simulink model "Multibody_2modules"  (R2024a)
settings: Solver=FixedStepAuto  StartTime=0.0  StopTime=TF  FixedStep=Ts  RelTol=1e-3
InitFcn:
  | close all
  | kinematics_2_modules
StopFcn:
  | results
model workspace: external: MATLAB File C:\Users\ricar\Documentos\MATLAB\OMNI_COUPLED\Coupled_SIMSCAPE_DataFile.m (data not in the file)
values from neighbouring files (symbols this model uses):
  eje_1 = 1    [kinematics_2_modules.m]    (also in kinematics_3_modules.m; kinematics_4modules.m; kinematics_front.m)
  eje_2 = 1    [kinematics_2_modules.m]    (also in kinematics_3_modules.m; kinematics_4modules.m; kinematics_front.m)
  eje_3 = 1    [kinematics_2_modules.m]    (also in kinematics_3_modules.m; kinematics_4modules.m; kinematics_front.m)
  eje_4 = 1    [kinematics_2_modules.m]    (also in kinematics_3_modules.m; kinematics_4modules.m; kinematics_front.m)
undefined symbols (not defined in the file or in its folder): fun_2mod_DK, smiData, X, Y, Z
libraries: sm_lib x362, nesl_utility x17, simulink x4, dspsigops x1
(part 1 of 6)
settings Model: Creator=ricar  LastModifiedBy=ricar
settings OptimizationCC: ReuseModelBlockBuffer=off
settings RTWCC: GPUComputeCapability=3.5
settings ExplorerConfigSet: InternalSimMechanicsExplorerSettings="<ExplorerConfiguration><canonicalview>planar_xy</canonicalview><AnimationSetting><BasePlaybackSpeed>1.0</BasePlaybackSpeed><PlaybackSpeedFactor>1.0</PlaybackSpeedFactor></AnimationSetting><TilePanel><TileInfo><Tiles Columns=\"1\" Count=\"1\" Rows=\"1\"><Column Weight=\"1\"/><Row Weight=\"1\"/><Tile Height=\"1\" Width=\"1\" X=\"0\" Y=\"0\"/></Tiles></TileInfo><SceneInfo><SceneViewer><BGColor><R>0.60000002384185791</R><G>0.60000002384185791</G><B>0.60000002384185791</B></BGColor><Camera><DoPerspective>off</DoPerspective><Position><X>1.22678896204454646</X><Y>1.20628904029276285</Y><Z>1.22678906359187656</Z></Position><Center><X>2.53292032547855483e-08</X><Y>-0.0204998964225804117</Y><Z>1.26876533262237912e-07</Z></Center><Up><X>-0.408248290463863073</X><Y>0.816496580927726145</Y><Z>-0.408248290463863073</Z></Up><ViewLimDist>1</ViewLimDist><YLim>1.38972711630507817</YLim><XLim>2.18495985507965074</XLim></Camera></SceneViewer></SceneInfo></TilePanel><MechEditorPanel><Cameras/><GfxPanelCameraMap/><VideoCreator><PlaybackSpeedRatio>1.0</PlaybackSpeedRatio><FrameRate>30</FrameRate><VideoFormat>Motion JPEG AVI</VideoFormat><FrameSize>auto</FrameSize></VideoCreator></MechEditorPanel></ExplorerConfiguration>"

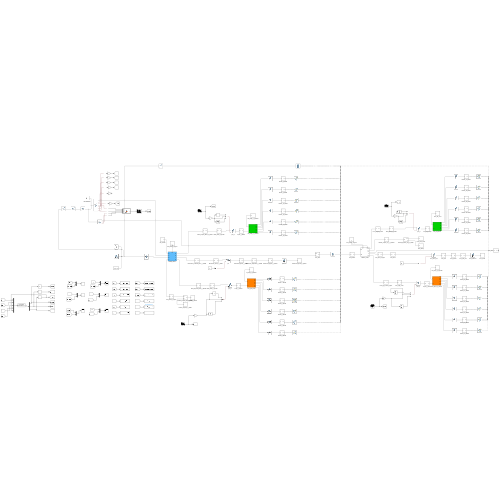
[thumbnail: Simulink's stored preview of the top-level diagram]
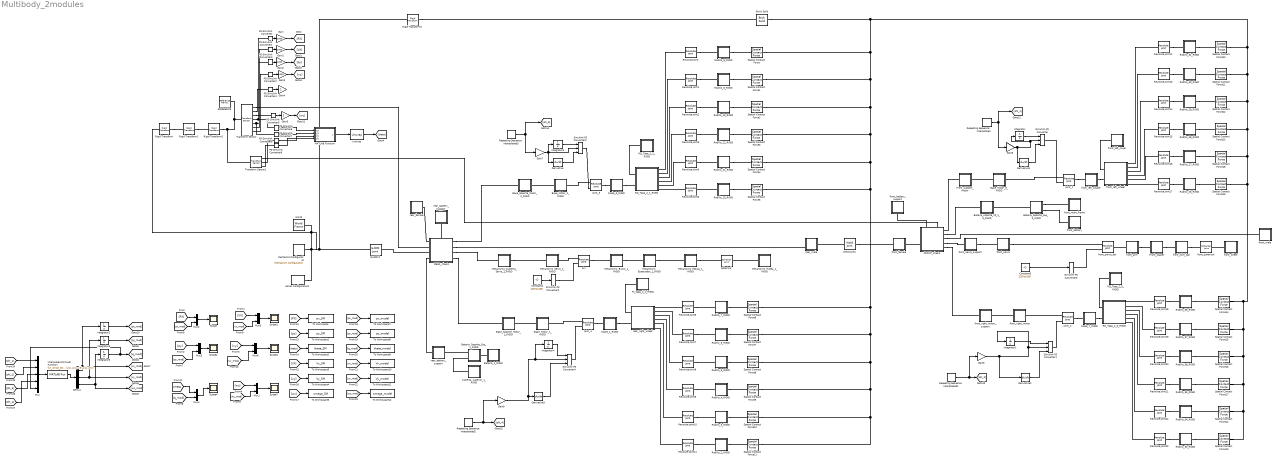
== system Multibody_2modules ==
  Base_Motor_1_RIGID : Subsystem
  Base_Motor_2_RIGID : Subsystem
  Base_Motor_6_RIGID : Subsystem
  Base_Soporte_Motor_1_RIGID : Subsystem
  Base_Soporte_Motor_2_RIGID : Subsystem
  Bateria_1_RIGID : Subsystem
  Bateria_Soporte_Sup_1_RIGID : Subsystem
  Bateria_Soporte_Sup_3_RIGID : Subsystem
  Bateria_soporte_Inf_1_3_RIGID : Subsystem
  Brick Solid : sm_lib/Body Elements/Brick Solid  BrickDimensions=[3 .002 3]  BrickDimensionsUnits=m  ExportEntireGeometry=on  InertiaType=CalculateFromGeometry  BasedOnType=Density  Density=1000  DensityUnits=kg/m^3  Mass=1  MassUnits=kg  CenterOfMass=[0 0 0]  CenterOfMassUnits=m  MomentsOfInertia=[1 1 1]  MomentsOfInertiaUnits=kg*m^2  ProductsOfInertia=[0 0 0]  ProductsOfInertiaUnits=kg*m^2  GraphicType=FromGeometry  MarkerShape=Sphere  MarkerSize=10  GraphicVisPropType=SimpleVisualProperties  GraphicDiffuseColor=[1 .6 .6]  GraphicOpacity=1  GraphicSpecularColor=[0.5 0.5 0.5 1.0]  GraphicAmbientColor=[0.15 0.15 0.15 1.0]  GraphicEmissiveColor=[0.0 0.0 0.0 1.0]  GraphicShininess=75  DoExposeReferenceFrame=on  SerializedFrames=<Frames/>
  Constant4 : Constant  Value=225*pi/180
  Constant5 : Constant  Value=225*pi/180
  Cople_1_RIGID : Subsystem
  Cople_3_RIGID : Subsystem
  Cople_7_RIGID : Subsystem
  Demux : Demux  Outputs=3
  Derivative{,1..3} (4 alike) : Derivative
  FRONT_chasis : Subsystem
      settings: PortSchema="{\"entries\":[{\"content\":{\"sides\":[{\"content\":{\"connectorIds\":[\"LConn1\",\"LConn2\"]},\"type\":\"ConnectorPlacement.EquallySpacedRectSide\",\"uuid\":\"2f193958-adda-4ec1-9c1e-8d18e10a43bf\"},{\"content\":{\"connectorIds\":[\"RConn1\",\"RConn2\",\"RConn3\",\"RConn4\",\"RConn5\"],\"side\":\"RIGHT\"},\"type\":\"ConnectorPlacement.EquallySpacedRectSide\",\"uuid\":\"9da4c68d-326e-4e0f-8b14-dbca64ff3e46\"},{\"content\":{\"connectorIds\":[\"LConn3\",\"LConn4\"],\"side\":\"TOP\"},\"type\":\"ConnectorPlacement.EquallySpacedRectSide\",\"uuid\":\"282e500d-48cf-43b0-8f8a-0690bc1d8b4d\"},{\"content\":{\"side\":\"BOTTOM\"},\"type\":\"ConnectorPlacement.EquallySpacedRectSide\",\"uuid\":\"3772ac25-9249-4303-a1a7-4471353d0084\"}]},\"type\":\"ConnectorPlacement.EquallySpacedConnector\",\"uuid\":\"3fae074b-7e70-469c-9f21-d7560799185b\"}],\"packageUris\":[\"http://schema.mathworks.com/mf0/Connector/R2020b\"],\"version\":\"1.0\"}"
  Front_spacer : Subsystem
  Front_support_motor : Subsystem
  Gain{,1..3} (4 alike) : Gain  Gain=1000
  Gain4 : Gain
  Gain5 : Gain
  Gain6 : Gain  Gain=eje_1
  Gain7 : Gain  Gain=eje_3
  Gain8 : Gain  Gain=eje_2
  Gain9 : Gain  Gain=eje_4
  Integrator{,1..6} (7 alike) : Integrator
  Interpreted MATLAB Function : MATLABFcn  MATLABFcn=fun_2mod_DK(u(1),u(2),u(3),u(4),u(5))
  MATLAB Function : MATLAB Function  TreatAsAtomicUnit=on
  Mecanismo_Brazo_1_RIGID : Subsystem
  Mecanismo_Cubierta_Servo_1_RIGID : Subsystem
  Mecanismo_Espaciador_1_RIGID : Subsystem
  Mecanismo_Rptula_1_RIGID : Subsystem
  Mecanismo_Rueda_1_RIGID : Subsystem
  Mecanismo_Servo_1_RIGID : Subsystem
  MechanismConfiguration : sm_lib/Utilities/Mechanism Configuration  UniformGravity=Constant  GravityVector=[0 -9.80665 0]  GravityVectorUnits=m/s^2  LinearizationDelta=0.001  JointModeTransitionNonlinearIterations=2
  Mux : Mux  Inputs=5
  Mux{1..6} (6 alike) : Mux  Inputs=2
  PS-Simulink Converter{,1..9} (10 alike) : nesl_utility/PS-Simulink Converter  PhysicalDomain=network_engine_domain  SubClassName=ps_output  LeftPortType=input  RightPortType=output  PseudoPeriodic=off  Frequencies=[]  VectorFormat=inherit  Unit=inherit  AffineConversion=off
  RD_Tapa_2_1_RIGID : Subsystem
  RD_Tapa_2_2_RIGID : Subsystem
  RD_Tapa_2_5_RIGID : Subsystem
  RD_Tapa_2_6_RIGID : Subsystem
  REAR_chasis : Subsystem
      settings: PortSchema="{\"entries\":[{\"content\":{\"sides\":[{\"content\":{\"connectorIds\":[\"LConn1\",\"LConn2\",\"LConn3\",\"LConn4\"]},\"type\":\"ConnectorPlacement.EquallySpacedRectSide\",\"uuid\":\"2f193958-adda-4ec1-9c1e-8d18e10a43bf\"},{\"content\":{\"connectorIds\":[\"RConn1\",\"RConn2\",\"RConn3\",\"RConn4\"],\"side\":\"RIGHT\"},\"type\":\"ConnectorPlacement.EquallySpacedRectSide\",\"uuid\":\"9da4c68d-326e-4e0f-8b14-dbca64ff3e46\"},{\"content\":{\"connectorIds\":[\"LConn5\"],\"side\":\"TOP\"},\"type\":\"ConnectorPlacement.EquallySpacedRectSide\",\"uuid\":\"282e500d-48cf-43b0-8f8a-0690bc1d8b4d\"}]},\"type\":\"ConnectorPlacement.EquallySpacedConnector\",\"uuid\":\"3fae074b-7e70-469c-9f21-d7560799185b\"}],\"packageUris\":[\"http://schema.mathworks.com/mf0/Connector/R2020b\"],\"version\":\"1.0\"}"
  REFERENCE : sm_lib/Frames and Transforms/Reference Frame
  RI_tapa_2_2_RIGID : Subsystem
  Repeating Sequence Interpolated : simulink/Sources/Repeating Sequence Interpolated  OutValues="1.5*[0  -1.49  -1.49  0   1.48  1.48   0  -2.96  -2.96  0  -1.46  -1.46 0]'"  TimeValues=[0 1 4 5 6 9 10 11 14 15 16 19 20]'  LookUpMeth=Interpolation-Use End Values  tsamp=0.0005  OutMin=[]  OutMax=[]  OutDataTypeStr=double  OutputDataTypeScalingMode=double  OutDataType=fixdt(0,8)  OutScaling=2^-10
  Repeating Sequence Interpolated1 : simulink/Sources/Repeating Sequence Interpolated  OutValues="1.5*[0  -1.49  -1.49  0  -4.44 -4.44   0  -2.96  -2.96  0  -1.46  -1.46 0]'"  TimeValues=[0 1 4 5 6 9 10 11 14 15 16 19 20]'  LookUpMeth=Interpolation-Use End Values  tsamp=0.0005  OutMin=[]  OutMax=[]  OutDataTypeStr=double  OutputDataTypeScalingMode=double  OutDataType=fixdt(0,8)  OutScaling=2^-10
  Repeating Sequence Interpolated2 : simulink/Sources/Repeating Sequence Interpolated  OutValues="1.5*[0   4.42   4.42  0  -1.48 -1.48   0   2.96   2.96  0  -1.49  -1.46 0]'"  TimeValues=[0 1 4 5 6 9 10 11 14 15 16 19 20]'  LookUpMeth=Interpolation-Use End Values  tsamp=0.0005  OutMin=[]  OutMax=[]  OutDataTypeStr=double  OutputDataTypeScalingMode=double  OutDataType=fixdt(0,8)  OutScaling=2^-10
  Repeating Sequence Interpolated3 : simulink/Sources/Repeating Sequence Interpolated  OutValues="1.5*[0   4.42   4.42  0   4.44  4.44   0   2.96   2.96  0  -1.46  -1.46 0]'"  TimeValues=[0 1 4 5 6 9 10 11 14 15 16 19 20]'  LookUpMeth=Interpolation-Use End Values  tsamp=0.0005  OutMin=[]  OutMax=[]  OutDataTypeStr=double  OutputDataTypeScalingMode=double  OutDataType=fixdt(0,8)  OutScaling=2^-10
  Revolute Joint{,1..23} (24 alike) : sm_lib/Joints/Revolute Joint  JointMode=Normal  CompositeWrenchDir=FollowerOnBase  CompositeWrenchFrame=BaseFrame  SenseConstraintForce=off  SenseConstraintTorque=off  SenseTotalForce=off  SenseTotalTorque=off  PositionTargetSpecify=off  PositionTargetPriority=High  PositionTargetValue=0  PositionTargetValueUnits=deg  VelocityTargetSpecify=off  VelocityTargetPriority=High  VelocityTargetValue=0  VelocityTargetValueUnits=deg/s  EquilibriumPosition=0  EquilibriumPositionUnits=deg  SpringStiffness=0  SpringStiffnessUnits=N*m/deg  DampingCoefficient=0  DampingCoefficientUnits=N*m/(deg/s)  LowerLimitSpecify=off  LowerLimitBound=-90  LowerLimitBoundUnits=deg  LowerLimitStiffness=1e4  LowerLimitStiffnessUnits=N*m/deg  LowerLimitDamping=10  LowerLimitDampingUnits=N*m/(deg/s)  LowerLimitTransitionRegionWidth=0.1  LowerLimitTransitionRegionWidthUnits=deg  UpperLimitSpecify=off  UpperLimitBound=90  UpperLimitBoundUnits=deg  UpperLimitStiffness=1e4  UpperLimitStiffnessUnits=N*m/deg  UpperLimitDamping=10  UpperLimitDampingUnits=N*m/(deg/s)  UpperLimitTransitionRegionWidth=0.1  UpperLimitTransitionRegionWidthUnits=deg  TorqueActuationMode=NoTorque  MotionActuationMode=ComputedMotion  SensePosition=off  SenseVelocity=off  SenseAcceleration=off  SenseTorqueForce=off  SenseLowerLimitTorqueForce=off  SenseUpperLimitTorqueForce=off
  Rigid Transform : sm_lib/Frames and Transforms/Rigid Transform  RotationMethod=StandardAxis  FollAlignAxisA=+X  BaseAlignAxisA=+Y  FollAlignAxisB=+Y  BaseAlignAxisB=+Z  RotationStandardAxis=+X  RotationAngle=-90  RotationAngleUnits=deg  RotationArbitraryAxis=[0 0 1]  RotationSequenceAxes=FollowerAxes  RotationSequence=XYX  RotationSequenceAngles=[0 0 0]  RotationSequenceAnglesUnits=deg  RotationMatrix=[1 0 0; 0 1 0; 0 0 1]  Quaternion=[1 0 0 0]  TranslationMethod=None  TranslationCartesianOffset=[0 0 0]  TranslationCartesianOffsetUnits=m  TranslationStandardAxis=+Z  TranslationStandardOffset=0  TranslationStandardOffsetUnits=m  TranslationROffset=0  TranslationROffsetUnits=m  TranslationThetaOffset=0  TranslationThetaOffsetUnits=deg  TranslationZOffset=0  TranslationZOffsetUnits=m
  Rigid Transform1 : sm_lib/Frames and Transforms/Rigid Transform  RotationMethod=StandardAxis  FollAlignAxisA=+X  BaseAlignAxisA=+Y  FollAlignAxisB=+Y  BaseAlignAxisB=+Z  RotationStandardAxis=+Z  RotationAngle=0  RotationAngleUnits=deg  RotationArbitraryAxis=[0 0 1]  RotationSequenceAxes=FollowerAxes  RotationSequence=XYX  RotationSequenceAngles=[0 0 0]  RotationSequenceAnglesUnits=deg  RotationMatrix=[1 0 0; 0 1 0; 0 0 1]  Quaternion=[1 0 0 0]  TranslationMethod=None  TranslationCartesianOffset=[0 0 0]  TranslationCartesianOffsetUnits=m  TranslationStandardAxis=+Z  TranslationStandardOffset=0  TranslationStandardOffsetUnits=m  TranslationROffset=0  TranslationROffsetUnits=m  TranslationThetaOffset=0  TranslationThetaOffsetUnits=deg  TranslationZOffset=0  TranslationZOffsetUnits=m
  Rigid Transform2 : sm_lib/Frames and Transforms/Rigid Transform  RotationMethod=None  FollAlignAxisA=+X  BaseAlignAxisA=+Y  FollAlignAxisB=+Y  BaseAlignAxisB=+Z  RotationStandardAxis=+Z  RotationAngle=0.0  RotationAngleUnits=deg  RotationArbitraryAxis=[0 0 1]  RotationSequenceAxes=FollowerAxes  RotationSequence=XYX  RotationSequenceAngles=[0 0 0]  RotationSequenceAnglesUnits=deg  RotationMatrix=[1 0 0; 0 1 0; 0 0 1]  Quaternion=[1 0 0 0]  TranslationMethod=StandardAxis  TranslationCartesianOffset=[0 0 0]  TranslationCartesianOffsetUnits=mm  TranslationStandardAxis=+X  TranslationStandardOffset=96-66  TranslationStandardOffsetUnits=mm  TranslationROffset=0  TranslationROffsetUnits=m  TranslationThetaOffset=0  TranslationThetaOffsetUnits=deg  TranslationZOffset=0  TranslationZOffsetUnits=m
  Rigid Transform3 : sm_lib/Frames and Transforms/Rigid Transform  RotationMethod=None  FollAlignAxisA=+X  BaseAlignAxisA=+Y  FollAlignAxisB=+Y  BaseAlignAxisB=+Z  RotationStandardAxis=+Z  RotationAngle=0  RotationAngleUnits=deg  RotationArbitraryAxis=[0 0 1]  RotationSequenceAxes=FollowerAxes  RotationSequence=XYX  RotationSequenceAngles=[0 0 0]  RotationSequenceAnglesUnits=deg  RotationMatrix=[1 0 0;0 1 0;0 0 1]  Quaternion=[1 0 0 0]  TranslationMethod=StandardAxis  TranslationCartesianOffset=[0 0 0]  TranslationCartesianOffsetUnits=m  TranslationStandardAxis=+Y  TranslationStandardOffset=-.0205  TranslationStandardOffsetUnits=m  TranslationROffset=0  TranslationROffsetUnits=m  TranslationThetaOffset=0  TranslationThetaOffsetUnits=deg  TranslationZOffset=0  TranslationZOffsetUnits=m
  Rodillo_10_RIGID : Subsystem
  Rodillo_11_RIGID : Subsystem
  Rodillo_12_RIGID : Subsystem
  Rodillo_13_RIGID : Subsystem
  Rodillo_26_RIGID : Subsystem
  Rodillo_27_RIGID : Subsystem
  Rodillo_28_RIGID : Subsystem
  Rodillo_29_RIGID : Subsystem
  Rodillo_2_RIGID : Subsystem
  Rodillo_30_RIGID : Subsystem
  Rodillo_31_RIGID : Subsystem
  Rodillo_33_RIGID : Subsystem
  Rodillo_34_RIGID : Subsystem
  Rodillo_35_RIGID : Subsystem
  Rodillo_36_RIGID : Subsystem
  Rodillo_37_RIGID : Subsystem
  Rodillo_38_RIGID : Subsystem
  Rodillo_3_RIGID : Subsystem
  Rodillo_4_RIGID : Subsystem
  Rodillo_5_RIGID : Subsystem
  Rodillo_6_RIGID : Subsystem
  Rodillo_7_RIGID : Subsystem
  Rodillo_8_RIGID : Subsystem
  Rodillo_9_RIGID : Subsystem
  Scope{,1..4,7} (6 alike) : Scope
  Simulink-PS Converter{,1,3..4} (4 alike) : nesl_utility/Simulink-PS Converter  PhysicalDomain=network_engine_domain  SubClassName=ps_input  LeftPortType=input  RightPortType=output  PseudoPeriodic=off  Frequencies=[]  NoiseDistribution=none  NoiseParameters=[]  Unit=1  AffineConversion=off  FilteringAndDerivatives=provide  SimscapeFilterOrder=1  InputFilterTimeConstant=0.001  UdotUserProvided=2
  Simulink-PS Converter2 : nesl_utility/Simulink-PS Converter  PhysicalDomain=network_engine_domain  SubClassName=ps_input  LeftPortType=input  RightPortType=output  PseudoPeriodic=off  Frequencies=[]  NoiseDistribution=none  NoiseParameters=[]  Unit=1  AffineConversion=off  FilteringAndDerivatives=zero  SimscapeFilterOrder=1  InputFilterTimeConstant=0.001  UdotUserProvided=0
  Simulink-PS Converter5 : nesl_utility/Simulink-PS Converter  PhysicalDomain=network_engine_domain  SubClassName=ps_input  LeftPortType=input  RightPortType=output  PseudoPeriodic=off  Frequencies=[]  NoiseDistribution=none  NoiseParameters=[]  Unit=1  AffineConversion=off  FilteringAndDerivatives=zero  SimscapeFilterOrder=1  InputFilterTimeConstant=0.001  UdotUserProvided=0
  SixDOF1 : sm_lib/Joints/6-DOF Joint  JointMode=Normal  CompositeWrenchDir=FollowerOnBase  CompositeWrenchFrame=BaseFrame  SenseConstraintForce=off  SenseConstraintTorque=off  SenseTotalForce=off  SenseTotalTorque=off  PxPositionTargetSpecify=off  PxPositionTargetPriority=High  PxPositionTargetValue=0  PxPositionTargetValueUnits=m  PxVelocityTargetSpecify=off  PxVelocityTargetPriority=High  PxVelocityTargetValue=0  PxVelocityTargetValueUnits=m/s  PxEquilibriumPosition=0  PxEquilibriumPositionUnits=m  PxSpringStiffness=0  PxSpringStiffnessUnits=N/m  PxDampingCoefficient=0  PxDampingCoefficientUnits=N/(m/s)  PxLowerLimitSpecify=off  PxLowerLimitBound=-1  PxLowerLimitBoundUnits=m  PxLowerLimitStiffness=1e6  PxLowerLimitStiffnessUnits=N/m  PxLowerLimitDamping=1e3  PxLowerLimitDampingUnits=N/(m/s)  PxLowerLimitTransitionRegionWidth=1e-4  PxLowerLimitTransitionRegionWidthUnits=m  PxUpperLimitSpecify=off  PxUpperLimitBound=1  PxUpperLimitBoundUnits=m  PxUpperLimitStiffness=1e6  PxUpperLimitStiffnessUnits=N/m  PxUpperLimitDamping=1e3  PxUpperLimitDampingUnits=N/(m/s)  PxUpperLimitTransitionRegionWidth=1e-4  PxUpperLimitTransitionRegionWidthUnits=m  PxTorqueActuationMode=NoTorque  PxMotionActuationMode=ComputedMotion  PxSensePosition=off  PxSenseVelocity=off  PxSenseAcceleration=off  PxSenseTorqueForce=off  PxSenseLowerLimitTorqueForce=off  PxSenseUpperLimitTorqueForce=off  PyPositionTargetSpecify=off  PyPositionTargetPriority=High  PyPositionTargetValue=0  PyPositionTargetValueUnits=m  PyVelocityTargetSpecify=off  PyVelocityTargetPriority=High  PyVelocityTargetValue=0  PyVelocityTargetValueUnits=m/s  PyEquilibriumPosition=0  PyEquilibriumPositionUnits=m  PySpringStiffness=0  PySpringStiffnessUnits=N/m  PyDampingCoefficient=0  PyDampingCoefficientUnits=N/(m/s)  PyLowerLimitSpecify=off  PyLowerLimitBound=-1  PyLowerLimitBoundUnits=m  PyLowerLimitStiffness=1e6  PyLowerLimitStiffnessUnits=N/m  PyLowerLimitDamping=1e3  PyLowerLimitDampingUnits=N/(m/s)  PyLowerLimitTransitionRegionWidth=1e-4  PyLowerLimitTransitionRegionWidthUnits=m  PyUpperLimitSpecify=off  PyUpperLimitBound=1  PyUpperLimitBoundUnits=m  PyUpperLimitStiffness=1e6  PyUpperLimitStiffnessUnits=N/m  PyUpperLimitDamping=1e3  PyUpperLimitDampingUnits=N/(m/s)  PyUpperLimitTransitionRegionWidth=1e-4  PyUpperLimitTransitionRegionWidthUnits=m  PyTorqueActuationMode=NoTorque  PyMotionActuationMode=ComputedMotion  PySensePosition=off  PySenseVelocity=off  PySenseAcceleration=off  PySenseTorqueForce=off  PySenseLowerLimitTorqueForce=off  PySenseUpperLimitTorqueForce=off  PzPositionTargetSpecify=off  PzPositionTargetPriority=High  PzPositionTargetValue=0  PzPositionTargetValueUnits=m  PzVelocityTargetSpecify=off  PzVelocityTargetPriority=High  PzVelocityTargetValue=0  PzVelocityTargetValueUnits=m/s  PzEquilibriumPosition=0  PzEquilibriumPositionUnits=m  PzSpringStiffness=0  PzSpringStiffnessUnits=N/m  PzDampingCoefficient=0  PzDampingCoefficientUnits=N/(m/s)  PzLowerLimitSpecify=off  PzLowerLimitBound=-1  PzLowerLimitBoundUnits=m  PzLowerLimitStiffness=1e6  PzLowerLimitStiffnessUnits=N/m  PzLowerLimitDamping=1e3  PzLowerLimitDampingUnits=N/(m/s)  PzLowerLimitTransitionRegionWidth=1e-4  PzLowerLimitTransitionRegionWidthUnits=m  PzUpperLimitSpecify=off  PzUpperLimitBound=1  PzUpperLimitBoundUnits=m  PzUpperLimitStiffness=1e6  PzUpperLimitStiffnessUnits=N/m  PzUpperLimitDamping=1e3  PzUpperLimitDampingUnits=N/(m/s)  PzUpperLimitTransitionRegionWidth=1e-4  PzUpperLimitTransitionRegionWidthUnits=m  PzTorqueActuationMode=NoTorque  PzMotionActuationMode=ComputedMotion  PzSensePosition=off  PzSenseVelocity=off  PzSenseAcceleration=off  PzSenseTorqueForce=off  PzSenseLowerLimitTorqueForce=off  PzSenseUpperLimitTorqueForce=off  SphPositionTargetSpecify=off  SphPositionTargetPriority=High  SphPositionTargetRotationMethod=None  SphPositionTargetFollAlignAxisA=+X  SphPositionTargetBaseAlignAxisA=+Y  SphPositionTargetFollAlignAxisB=+Y  SphPositionTargetBaseAlignAxisB=+Z  SphPositionTargetRotationStandardAxis=+Z  SphPositionTargetRotationAngle=0.0  SphPositionTargetRotationAngleUnits=deg  SphPositionTargetRotationArbitraryAxis=[0 0 1]  SphPositionTargetRotationSequenceAxes=FollowerAxes  SphPositionTargetRotationSequence=XYX  SphPositionTargetRotationSequenceAngles=[0 0 0]  SphPositionTargetRotationSequenceAnglesUnits=deg  SphPositionTargetRotationMatrix=[1 0 0; 0 1 0; 0 0 1]  SphPositionTargetQuaternion=[1 0 0 0]  SphVelocityTargetSpecify=off  SphVelocityTargetPriority=High  SphVelocityTargetValue=[0 0 0]  SphVelocityTargetValueUnits=deg/s  SphVelocityTargetInFollowerFrame=on  SphEqPosRotationMethod=None  SphEqPosFollAlignAxisA=+X  SphEqPosBaseAlignAxisA=+Y  SphEqPosFollAlignAxisB=+Y  SphEqPosBaseAlignAxisB=+Z  SphEqPosRotationStandardAxis=+Z  SphEqPosRotationAngle=0.0  SphEqPosRotationAngleUnits=deg  SphEqPosRotationArbitraryAxis=[0 0 1]  SphEqPosRotationSequenceAxes=FollowerAxes  SphEqPosRotationSequence=XYX  SphEqPosRotationSequenceAngles=[0 0 0]  SphEqPosRotationSequenceAnglesUnits=deg  SphEqPosRotationMatrix=[1 0 0; 0 1 0; 0 0 1]  SphEqPosQuaternion=[1 0 0 0]  SphSpringStiffness=0  SphSpringStiffnessUnits=N*m/deg  SphDampingCoefficient=0  SphDampingCoefficientUnits=N*m/(deg/s)  SphLowerLimitSpecify=off  SphLowerLimitBound=15  SphLowerLimitBoundUnits=deg  SphLowerLimitStiffness=1e4  SphLowerLimitStiffnessUnits=N*m/deg  SphLowerLimitDamping=10  SphLowerLimitDampingUnits=N*m/(deg/s)  SphLowerLimitTransitionRegionWidth=0.1  SphLowerLimitTransitionRegionWidthUnits=deg  SphUpperLimitSpecify=off  SphUpperLimitBound=45  SphUpperLimitBoundUnits=deg  SphUpperLimitStiffness=1e4  SphUpperLimitStiffnessUnits=N*m/deg  SphUpperLimitDamping=10  SphUpperLimitDampingUnits=N*m/(deg/s)  SphUpperLimitTransitionRegionWidth=0.1  SphUpperLimitTransitionRegionWidthUnits=deg  SphTorqueActuationMode=NoTorque  SphActuateTorqueX=off  SphActuateTorqueY=off  SphActuateTorqueZ=off  SphActuateTorque=off  SphActuationFrame=BaseFrame  SphSensePosition=off  SphSenseVelocityX=off  SphSenseVelocityY=off  SphSenseVelocityZ=off  SphSenseVelocity=off  SphSenseAccelerationX=off  SphSenseAccelerationY=off  SphSenseAccelerationZ=off  SphSenseAcceleration=off  SphSenseLowerLimitTorqueMag=off  SphSenseUpperLimitTorqueMag=off  SphSensingFrame=FollowerFrame
  Solver Configuration1 : nesl_utility/Solver Configuration  PhysicalDomain=network_engine_domain  SubClassName=solver  LeftPortType=input  RightPortType=generic  Tones=[]  Harmonics=[]  SimulateNoise=off  Profile=off  UseLocalSampling=off  EnableSwitchedLinearOptims=on  FrequencyDomain=off  UseCCode=off  RelTol=0.001  AbsTol=0.001  MinStep=1e-09  ToWorkspace=off  RevertToSquareIcSolve=off  NumHomotopyIterations=100  PhasorMode=off  PhasorModeNumHarmonics=1  ConsistencySolver=NEWTON_XTOL_AFTER_FTOL  IndexReductionMethod=DerivativeReplacement  DoDC=off  ResidualTolerance=1e-09  ConsistencyTolSource=GLOBAL  ConsistencyAbsTol=0.001  ConsistencyRelTol=0.001  ConsistencyTolFactor=0.001  UseLocalSolver=off  LocalSolverChoice=NE_BACKWARD_EULER_ADVANCER  ResolveIndetEquations=on  FunctionEvalNumThread=1  LocalSolverSampleTime=0.001  DoFixedCost=off  MaxNonlinIter=3  MaxModeIter=2  ComputeImpulses=off  ImpulseIterations=2  LinearAlgebra=auto  LinearAlgebraNumThread=0  EquationFormulation=NE_TIME_EF  DelaysMemoryBudget=1024  AutomaticFiltering=on  FilteringTimeConstant=0.001  PartitionStorageMethod=AS_NEEDED  PartitionMemoryBudget=1024  PartitionMethod=ROBUST  MultibodyUseLocalSolver=off  MultibodyLocalSolverChoice=ODE1  MultibodyLocalSolverSampleTime=0.001
  Spatial Contact Force{,1..23} (24 alike) : sm_lib/Forces and Torques/Spatial Contact Force  NormalForceType=SmoothSpringDamper  NormalStiffness=1e6  NormalStiffnessUnits=N/m  NormalDamping=1e3  NormalDampingUnits=N/(m/s)  NormalTransitionRegionWidth=1e-4  NormalTransitionRegionWidthUnits=m  FrictionType=SmoothStickSlip  CoefficientOfStaticFriction=0.5  CoefficientOfDynamicFriction=0.3  FrictionalCriticalVelocity=1e-3  FrictionalCriticalVelocityUnits=m/s  SenseContactSignal=off  SensePenetrationDepth=off  SenseSeparationDistance=off  SenseNormalForceMagnitude=off  SenseFrictionalForceMagnitude=off  SenseNormalVelocity=off  SenseTangentialVelocity=off  SenseContactBaseRotation=off  SenseContactBaseTranslation=off  SenseContactFollowerRotation=off  SenseContactFollowerTranslation=off  ZeroCrossDetectContactStartAndEnd=off
  Spherical : sm_lib/Joints/Spherical Joint  JointMode=Normal  CompositeWrenchDir=FollowerOnBase  CompositeWrenchFrame=BaseFrame  SenseConstraintForce=off  SenseConstraintTorque=off  SenseTotalForce=off  SenseTotalTorque=off  PositionTargetSpecify=off  PositionTargetPriority=Low  PositionTargetRotationMethod=ArbitraryAxis  PositionTargetFollAlignAxisA=+X  PositionTargetBaseAlignAxisA=+Y  PositionTargetFollAlignAxisB=+Y  PositionTargetBaseAlignAxisB=+Z  PositionTargetRotationStandardAxis=+Z  PositionTargetRotationAngle=smiData.SphericalJoint(1).S.Pos.Angle  PositionTargetRotationAngleUnits=deg  PositionTargetRotationArbitraryAxis=smiData.SphericalJoint(1).S.Pos.Axis  PositionTargetRotationSequenceAxes=FollowerAxes  PositionTargetRotationSequence=XYX  PositionTargetRotationSequenceAngles=[0 0 0]  PositionTargetRotationSequenceAnglesUnits=deg  PositionTargetRotationMatrix=[1 0 0; 0 1 0; 0 0 1]  PositionTargetQuaternion=[1 0 0 0]  VelocityTargetSpecify=off  VelocityTargetPriority=High  VelocityTargetValue=[0 0 0]  VelocityTargetValueUnits=deg/s  VelocityTargetInFollowerFrame=on  EqPosRotationMethod=None  EqPosFollAlignAxisA=+X  EqPosBaseAlignAxisA=+Y  EqPosFollAlignAxisB=+Y  EqPosBaseAlignAxisB=+Z  EqPosRotationStandardAxis=+Z  EqPosRotationAngle=0.0  EqPosRotationAngleUnits=deg  EqPosRotationArbitraryAxis=[0 0 1]  EqPosRotationSequenceAxes=FollowerAxes  EqPosRotationSequence=XYX  EqPosRotationSequenceAngles=[0 0 0]  EqPosRotationSequenceAnglesUnits=deg  EqPosRotationMatrix=[1 0 0; 0 1 0; 0 0 1]  EqPosQuaternion=[1 0 0 0]  SpringStiffness=0  SpringStiffnessUnits=N*m/deg  DampingCoefficient=0  DampingCoefficientUnits=N*m/(deg/s)  LowerLimitSpecify=off  LowerLimitBound=15  LowerLimitBoundUnits=deg  LowerLimitStiffness=1e4  LowerLimitStiffnessUnits=N*m/deg  LowerLimitDamping=10  LowerLimitDampingUnits=N*m/(deg/s)  LowerLimitTransitionRegionWidth=0.1  LowerLimitTransitionRegionWidthUnits=deg  UpperLimitSpecify=off  UpperLimitBound=45  UpperLimitBoundUnits=deg  UpperLimitStiffness=1e4  UpperLimitStiffnessUnits=N*m/deg  UpperLimitDamping=10  UpperLimitDampingUnits=N*m/(deg/s)  UpperLimitTransitionRegionWidth=0.1  UpperLimitTransitionRegionWidthUnits=deg  TorqueActuationMode=NoTorque  ActuateTorqueX=off  ActuateTorqueY=off  ActuateTorqueZ=off  ActuateTorque=off  ActuationFrame=BaseFrame  SensePosition=off  SenseVelocityX=off  SenseVelocityY=off  SenseVelocityZ=off  SenseVelocity=off  SenseAccelerationX=off  SenseAccelerationY=off  SenseAccelerationZ=off  SenseAcceleration=off  SenseLowerLimitTorqueMag=off  SenseUpperLimitTorqueMag=off  SensingFrame=FollowerFrame
  To Workspace : ToWorkspace  VariableName=px_SM  SaveFormat=Structure  SampleTime=-1
      settings: Save2DSignal=2-D array (concatenate along first dimension)
  To Workspace1 : ToWorkspace  VariableName=py_SM  SaveFormat=Structure  SampleTime=-1
      settings: Save2DSignal=2-D array (concatenate along first dimension)
  To Workspace10 : ToWorkspace  VariableName=Vx_model  SaveFormat=Structure  SampleTime=-1
      settings: Save2DSignal=2-D array (concatenate along first dimension)
  To Workspace11 : ToWorkspace  VariableName=Vy_model  SaveFormat=Structure  SampleTime=-1
      settings: Save2DSignal=2-D array (concatenate along first dimension)
  To Workspace12 : ToWorkspace  VariableName=omega_model  SaveFormat=Structure  SampleTime=-1
      settings: Save2DSignal=2-D array (concatenate along first dimension)
  To Workspace2 : ToWorkspace  VariableName=theta_SM  SaveFormat=Structure  SampleTime=-1
      settings: Save2DSignal=2-D array (concatenate along first dimension)
  To Workspace3 : ToWorkspace  VariableName=Vx_SM  SaveFormat=Structure  SampleTime=-1
      settings: Save2DSignal=2-D array (concatenate along first dimension)
  To Workspace4 : ToWorkspace  VariableName=Vy_SM  SaveFormat=Structure  SampleTime=-1
      settings: Save2DSignal=2-D array (concatenate along first dimension)
  To Workspace5 : ToWorkspace  VariableName=omega_SM  SaveFormat=Structure  SampleTime=-1
      settings: Save2DSignal=2-D array (concatenate along first dimension)
  To Workspace7 : ToWorkspace  VariableName=px_model  SaveFormat=Structure  SampleTime=-1
      settings: Save2DSignal=2-D array (concatenate along first dimension)
  To Workspace8 : ToWorkspace  VariableName=py_model  SaveFormat=Structure  SampleTime=-1
      settings: Save2DSignal=2-D array (concatenate along first dimension)
  To Workspace9 : ToWorkspace  VariableName=theta_model  SaveFormat=Structure  SampleTime=-1
      settings: Save2DSignal=2-D array (concatenate along first dimension)
  Transform Sensor : sm_lib/Frames and Transforms/Transform Sensor  MeasurementFrame=Base  RotationSequence=XYX  SenseAngle=on  SenseAxis=off  SenseQ=off  SenseR=off  SenseRotationSequence=off  SenseOmegaX=off  SenseOmegaY=off  SenseOmegaZ=on  SenseOmega=off  SenseQDot=off  SenseRDot=off  SenseRotationSequenceDot=off  SenseAlphaX=off  SenseAlphaY=off  SenseAlphaZ=off  SenseAlpha=off  SenseQDDot=off  SenseRDDot=off  SenseX=on  SenseY=on  SenseZ=off  SenseXYZ=off  SenseRad=off  SenseAzim=off  SenseDist=off  SenseInc=off  SenseXDot=on  SenseYDot=on  SenseZDot=off  SenseXYZDot=off  SenseRadDot=off  SenseAzimDot=off  SenseDistDot=off  SenseIncDot=off  SenseXDDot=off  SenseYDDot=off  SenseZDDot=off  SenseXYZDDot=off  SenseRadDDot=off  SenseAzimDDot=off  SenseDistDDot=off  SenseIncDDot=off
  Transform Sensor1 : sm_lib/Frames and Transforms/Transform Sensor  MeasurementFrame=Base  RotationSequence=XYX  SenseAngle=off  SenseAxis=off  SenseQ=off  SenseR=off  SenseRotationSequence=off  SenseOmegaX=off  SenseOmegaY=off  SenseOmegaZ=off  SenseOmega=off  SenseQDot=off  SenseRDot=off  SenseRotationSequenceDot=off  SenseAlphaX=off  SenseAlphaY=off  SenseAlphaZ=off  SenseAlpha=off  SenseQDDot=off  SenseRDDot=off  SenseX=on  SenseY=on  SenseZ=off  SenseXYZ=off  SenseRad=off  SenseAzim=off  SenseDist=off  SenseInc=off  SenseXDot=off  SenseYDot=off  SenseZDot=off  SenseXYZDot=off  SenseRadDot=off  SenseAzimDot=off  SenseDistDot=off  SenseIncDot=off  SenseXDDot=off  SenseYDDot=off  SenseZDDot=off  SenseXYZDDot=off  SenseRadDDot=off  SenseAzimDDot=off  SenseDistDDot=off  SenseIncDDot=off
  Unwrap : dspsigops/Unwrap  tol=pi  InputProcessing=Columns as channels (frame based)  running=off
  Weld Joint1 : sm_lib/Joints/Weld Joint  JointMode=Normal  CompositeWrenchDir=FollowerOnBase  CompositeWrenchFrame=BaseFrame  SenseConstraintForce=off  SenseConstraintTorque=off  SenseTotalForce=off  SenseTotalTorque=off
  World : sm_lib/Frames and Transforms/World Frame
  cubierta_superior_1_RIGID : Subsystem
  front_arm : Subsystem
  front_battery : Subsystem
  front_battery_support : Subsystem
      settings: PortSchema="{\"entries\":[{\"content\":{\"sides\":[{\"content\":{\"connectorIds\":[]},\"type\":\"ConnectorPlacement.EquallySpacedRectSide\",\"uuid\":\"43eea88b-bd11-4c8a-9d6e-a076a733ec0a\"},{\"content\":{\"connectorIds\":[],\"side\":\"RIGHT\"},\"type\":\"ConnectorPlacement.EquallySpacedRectSide\",\"uuid\":\"0041fe48-15ee-4c36-9983-1d06526567a7\"},{\"content\":{\"connectorIds\":[],\"side\":\"TOP\"},\"type\":\"ConnectorPlacement.EquallySpacedRectSide\",\"uuid\":\"107a4c7a-824b-4d0c-9fc5-365ed2c75f27\"},{\"content\":{\"connectorIds\":[\"RConn1\"],\"side\":\"BOTTOM\"},\"type\":\"ConnectorPlacement.EquallySpacedRectSide\",\"uuid\":\"9e5ecfdb-895f-4943-b8dd-167b69fc8e9b\"}]},\"type\":\"ConnectorPlacement.EquallySpacedConnector\",\"uuid\":\"72f4945d-6267-4dc9-8f2c-fa0eb7282087\"}],\"packageUris\":[\"http://schema.mathworks.com/mf0/Connector/R2020b\"],\"version\":\"1.0\"}"
  front_female : Subsystem
  front_joint_ball : Subsystem
  front_left_couple : Subsystem
  front_left_cover : Subsystem
  front_left_wheel : Subsystem
  front_main_frame : Subsystem
  front_male : Subsystem
      settings: PortSchema="{\"entries\":[{\"content\":{\"sides\":[{\"content\":{},\"type\":\"ConnectorPlacement.EquallySpacedRectSide\",\"uuid\":\"43eea88b-bd11-4c8a-9d6e-a076a733ec0a\"},{\"content\":{\"side\":\"RIGHT\"},\"type\":\"ConnectorPlacement.EquallySpacedRectSide\",\"uuid\":\"0041fe48-15ee-4c36-9983-1d06526567a7\"},{\"content\":{\"connectorIds\":[\"LConn1\"],\"side\":\"TOP\"},\"type\":\"ConnectorPlacement.EquallySpacedRectSide\",\"uuid\":\"107a4c7a-824b-4d0c-9fc5-365ed2c75f27\"},{\"content\":{\"connectorIds\":[\"RConn1\"],\"side\":\"BOTTOM\"},\"type\":\"ConnectorPlacement.EquallySpacedRectSide\",\"uuid\":\"88e7dade-3fbf-49af-95f0-217e5cb73aaf\"}]},\"type\":\"ConnectorPlacement.EquallySpacedConnector\",\"uuid\":\"72f4945d-6267-4dc9-8f2c-fa0eb7282087\"}],\"packageUris\":[\"http://schema.mathworks.com/mf0/Connector/R2020b\"],\"version\":\"1.0\"}"
  front_right_motor : Subsystem
  front_rigth_motor_support : Subsystem
  front_servo : Subsystem
  front_servo_act : sm_lib/Joints/Revolute Joint  JointMode=Normal  CompositeWrenchDir=FollowerOnBase  CompositeWrenchFrame=BaseFrame  SenseConstraintForce=off  SenseConstraintTorque=off  SenseTotalForce=off  SenseTotalTorque=off  PositionTargetSpecify=on  PositionTargetPriority=Low  PositionTargetValue=smiData.RevoluteJoint(14).Rz.Pos  PositionTargetValueUnits=deg  VelocityTargetSpecify=off  VelocityTargetPriority=High  VelocityTargetValue=0  VelocityTargetValueUnits=deg/s  EquilibriumPosition=0  EquilibriumPositionUnits=deg  SpringStiffness=0  SpringStiffnessUnits=N*m/deg  DampingCoefficient=0  DampingCoefficientUnits=N*m/(deg/s)  LowerLimitSpecify=off  LowerLimitBound=-90  LowerLimitBoundUnits=deg  LowerLimitStiffness=1e4  LowerLimitStiffnessUnits=N*m/deg  LowerLimitDamping=10  LowerLimitDampingUnits=N*m/(deg/s)  LowerLimitTransitionRegionWidth=0.1  LowerLimitTransitionRegionWidthUnits=deg  UpperLimitSpecify=off  UpperLimitBound=90  UpperLimitBoundUnits=deg  UpperLimitStiffness=1e4  UpperLimitStiffnessUnits=N*m/deg  UpperLimitDamping=10  UpperLimitDampingUnits=N*m/(deg/s)  UpperLimitTransitionRegionWidth=0.1  UpperLimitTransitionRegionWidthUnits=deg  TorqueActuationMode=ComputedTorque  MotionActuationMode=InputMotion  SensePosition=off  SenseVelocity=off  SenseAcceleration=off  SenseTorqueForce=off  SenseLowerLimitTorqueForce=off  SenseUpperLimitTorqueForce=off
  front_servo_support : Subsystem
  front_spherical : sm_lib/Joints/Spherical Joint  JointMode=Normal  CompositeWrenchDir=FollowerOnBase  CompositeWrenchFrame=BaseFrame  SenseConstraintForce=off  SenseConstraintTorque=off  SenseTotalForce=off  SenseTotalTorque=off  PositionTargetSpecify=on  PositionTargetPriority=Low  PositionTargetRotationMethod=ArbitraryAxis  PositionTargetFollAlignAxisA=+X  PositionTargetBaseAlignAxisA=+Y  PositionTargetFollAlignAxisB=+Y  PositionTargetBaseAlignAxisB=+Z  PositionTargetRotationStandardAxis=+Z  PositionTargetRotationAngle=smiData.SphericalJoint(2).S.Pos.Angle  PositionTargetRotationAngleUnits=deg  PositionTargetRotationArbitraryAxis=smiData.SphericalJoint(2).S.Pos.Axis  PositionTargetRotationSequenceAxes=FollowerAxes  PositionTargetRotationSequence=XYX  PositionTargetRotationSequenceAngles=[0 0 0]  PositionTargetRotationSequenceAnglesUnits=deg  PositionTargetRotationMatrix=[1 0 0; 0 1 0; 0 0 1]  PositionTargetQuaternion=[1 0 0 0]  VelocityTargetSpecify=off  VelocityTargetPriority=High  VelocityTargetValue=[0 0 0]  VelocityTargetValueUnits=deg/s  VelocityTargetInFollowerFrame=on  EqPosRotationMethod=None  EqPosFollAlignAxisA=+X  EqPosBaseAlignAxisA=+Y  EqPosFollAlignAxisB=+Y  EqPosBaseAlignAxisB=+Z  EqPosRotationStandardAxis=+Z  EqPosRotationAngle=0.0  EqPosRotationAngleUnits=deg  EqPosRotationArbitraryAxis=[0 0 1]  EqPosRotationSequenceAxes=FollowerAxes  EqPosRotationSequence=XYX  EqPosRotationSequenceAngles=[0 0 0]  EqPosRotationSequenceAnglesUnits=deg  EqPosRotationMatrix=[1 0 0; 0 1 0; 0 0 1]  EqPosQuaternion=[1 0 0 0]  SpringStiffness=0  SpringStiffnessUnits=N*m/deg  DampingCoefficient=0  DampingCoefficientUnits=N*m/(deg/s)  LowerLimitSpecify=off  LowerLimitBound=15  LowerLimitBoundUnits=deg  LowerLimitStiffness=1e4  LowerLimitStiffnessUnits=N*m/deg  LowerLimitDamping=10  LowerLimitDampingUnits=N*m/(deg/s)  LowerLimitTransitionRegionWidth=0.1  LowerLimitTransitionRegionWidthUnits=deg  UpperLimitSpecify=off  UpperLimitBound=45  UpperLimitBoundUnits=deg  UpperLimitStiffness=1e4  UpperLimitStiffnessUnits=N*m/deg  UpperLimitDamping=10  UpperLimitDampingUnits=N*m/(deg/s)  UpperLimitTransitionRegionWidth=0.1  UpperLimitTransitionRegionWidthUnits=deg  TorqueActuationMode=NoTorque  ActuateTorqueX=off  ActuateTorqueY=off  ActuateTorqueZ=off  ActuateTorque=off  ActuationFrame=BaseFrame  SensePosition=off  SenseVelocityX=off  SenseVelocityY=off  SenseVelocityZ=off  SenseVelocity=off  SenseAccelerationX=off  SenseAccelerationY=off  SenseAccelerationZ=off  SenseAcceleration=off  SenseLowerLimitTorqueMag=off  SenseUpperLimitTorqueMag=off  SensingFrame=FollowerFrame
  front_wheel : Subsystem
  joint_{1..4} (4 alike) : sm_lib/Joints/Revolute Joint  JointMode=Normal  CompositeWrenchDir=FollowerOnBase  CompositeWrenchFrame=BaseFrame  SenseConstraintForce=off  SenseConstraintTorque=off  SenseTotalForce=off  SenseTotalTorque=off  PositionTargetSpecify=off  PositionTargetPriority=High  PositionTargetValue=0  PositionTargetValueUnits=deg  VelocityTargetSpecify=off  VelocityTargetPriority=High  VelocityTargetValue=0  VelocityTargetValueUnits=deg/s  EquilibriumPosition=0  EquilibriumPositionUnits=deg  SpringStiffness=0  SpringStiffnessUnits=N*m/deg  DampingCoefficient=0  DampingCoefficientUnits=N*m/(deg/s)  LowerLimitSpecify=off  LowerLimitBound=-90  LowerLimitBoundUnits=deg  LowerLimitStiffness=1e4  LowerLimitStiffnessUnits=N*m/deg  LowerLimitDamping=10  LowerLimitDampingUnits=N*m/(deg/s)  LowerLimitTransitionRegionWidth=0.1  LowerLimitTransitionRegionWidthUnits=deg  UpperLimitSpecify=off  UpperLimitBound=90  UpperLimitBoundUnits=deg  UpperLimitStiffness=1e4  UpperLimitStiffnessUnits=N*m/deg  UpperLimitDamping=10  UpperLimitDampingUnits=N*m/(deg/s)  UpperLimitTransitionRegionWidth=0.1  UpperLimitTransitionRegionWidthUnits=deg  TorqueActuationMode=ComputedTorque  MotionActuationMode=InputMotion  SensePosition=off  SenseVelocity=off  SenseAcceleration=off  SenseTorqueForce=off  SenseLowerLimitTorqueForce=off  SenseUpperLimitTorqueForce=off
  pin : sm_lib/Joints/Revolute Joint  JointMode=Normal  CompositeWrenchDir=FollowerOnBase  CompositeWrenchFrame=BaseFrame  SenseConstraintForce=off  SenseConstraintTorque=off  SenseTotalForce=off  SenseTotalTorque=off  PositionTargetSpecify=on  PositionTargetPriority=Low  PositionTargetValue=225  PositionTargetValueUnits=deg  VelocityTargetSpecify=off  VelocityTargetPriority=High  VelocityTargetValue=0  VelocityTargetValueUnits=deg/s  EquilibriumPosition=0  EquilibriumPositionUnits=deg  SpringStiffness=0  SpringStiffnessUnits=N*m/deg  DampingCoefficient=0  DampingCoefficientUnits=N*m/(deg/s)  LowerLimitSpecify=off  LowerLimitBound=-90  LowerLimitBoundUnits=deg  LowerLimitStiffness=1e4  LowerLimitStiffnessUnits=N*m/deg  LowerLimitDamping=10  LowerLimitDampingUnits=N*m/(deg/s)  LowerLimitTransitionRegionWidth=0.1  LowerLimitTransitionRegionWidthUnits=deg  UpperLimitSpecify=off  UpperLimitBound=90  UpperLimitBoundUnits=deg  UpperLimitStiffness=1e4  UpperLimitStiffnessUnits=N*m/deg  UpperLimitDamping=10  UpperLimitDampingUnits=N*m/(deg/s)  UpperLimitTransitionRegionWidth=0.1  UpperLimitTransitionRegionWidthUnits=deg  TorqueActuationMode=ComputedTorque  MotionActuationMode=InputMotion  SensePosition=off  SenseVelocity=off  SenseAcceleration=off  SenseTorqueForce=off  SenseLowerLimitTorqueForce=off  SenseUpperLimitTorqueForce=off
  rear_battery_support : Subsystem
  rear_battery_supppor : Subsystem
      settings: PortSchema="{\"entries\":[{\"content\":{\"sides\":[{\"content\":{\"connectorIds\":[]},\"type\":\"ConnectorPlacement.EquallySpacedRectSide\",\"uuid\":\"49fd6699-5409-4602-99e4-a32cb97dd5d0\"},{\"content\":{\"connectorIds\":[],\"side\":\"RIGHT\"},\"type\":\"ConnectorPlacement.EquallySpacedRectSide\",\"uuid\":\"b7f73f1c-1ff2-40c9-b6ab-0cb0d23d3350\"},{\"content\":{\"connectorIds\":[],\"side\":\"TOP\"},\"type\":\"ConnectorPlacement.EquallySpacedRectSide\",\"uuid\":\"25483bf1-1407-4122-84af-ca086ca47459\"},{\"content\":{\"connectorIds\":[\"RConn1\"],\"side\":\"BOTTOM\"},\"type\":\"ConnectorPlacement.EquallySpacedRectSide\",\"uuid\":\"19056d6d-ce15-4019-9505-0883534a59fe\"}]},\"type\":\"ConnectorPlacement.EquallySpacedConnector\",\"uuid\":\"8172ee3c-b33e-4346-8b95-395c4a40ccc2\"}],\"packageUris\":[\"http://schema.mathworks.com/mf0/Connector/R2020b\"],\"version\":\"1.0\"}"
  rear_female : Subsystem
  rear_male : Subsystem
  rear_right_wheel : Subsystem
  wires:
  Integrator/1 -> Simulink-PS Converter/1
  Integrator1/1 -> Simulink-PS Converter1/1
  Integrator3/1 -> Simulink-PS Converter3/1
  Integrator4/1 -> Simulink-PS Converter4/1
  Constant4/1 -> Simulink-PS Converter2/1
  Constant5/1 -> Simulink-PS Converter5/1
  [vx_mod] -> To Workspace10/1
  [theta] -> Mux4/1
  [vy_mod] -> Mux6/2
  Interpreted MATLAB Function/1 -> Demux/1
  [vy_mod] -> To Workspace11/1
  [VX] -> To Workspace3/1
  [wz] -> To Workspace5/1
  [px_mod] -> To Workspace7/1
  Mux4/1 -> Scope4/1
  [vy] -> Mux6/1
  [px_mod] -> Mux2/2
  Integrator6/1 -> Mux/5, [q_mod]
  [py_mod] -> Mux3/2
  [py] -> Mux3/1
  [py] -> To Workspace1/1
  Mux3/1 -> Scope2/1
  [vx_mod] -> Mux5/2
  [theta] -> To Workspace2/1
  Mux1/1 -> Scope7/1
  Mux2/1 -> Scope/1
  [PX] -> To Workspace/1
  [wz_mod] -> Mux1/2
  [vy] -> To Workspace4/1
  [py_mod] -> To Workspace8/1
  [PX] -> Mux2/1
  Mux5/1 -> Scope1/1
  Mux6/1 -> Scope3/1
  Demux/3 -> Integrator6/1, [wz_mod]
  [wz] -> Mux1/1
  [q_mod] -> To Workspace9/1
  Demux/2 -> Integrator5/1, [vy_mod]
  [wz_mod] -> To Workspace12/1
  Integrator5/1 -> [py_mod]
  Mux/1 -> Interpreted MATLAB Function/1
  Demux/1 -> Integrator2/1, [vx_mod]
  [q_mod] -> Mux4/2
  Integrator2/1 -> [px_mod]
  Gain3/1 -> [vy]
  Gain5/1 -> [wz]
  PS-Simulink Converter3/1 -> Gain2/1
  PS-Simulink Converter1/1 -> Gain1/1
  PS-Simulink Converter5/1 -> Gain5/1
  Gain1/1 -> [VX]
  PS-Simulink Converter4/1 -> Gain4/1
  PS-Simulink Converter/1 -> Gain/1
  PS-Simulink Converter2/1 -> Gain3/1
  Gain/1 -> [PX]
  Gain2/1 -> [py]
  [VX] -> Mux5/1
  Gain6/1 -> Derivative1/1, Simulink-PS Converter/2, Integrator/1
  Gain7/1 -> Derivative/1, Integrator3/1, Simulink-PS Converter3/2
  Derivative/1 -> Simulink-PS Converter3/3
  Derivative1/1 -> Simulink-PS Converter/3
  Derivative2/1 -> Simulink-PS Converter1/3
  Derivative3/1 -> Simulink-PS Converter4/3
  Gain8/1 -> Derivative2/1, Simulink-PS Converter1/2, Integrator1/1
  Gain9/1 -> Simulink-PS Converter4/2, Integrator4/1, Derivative3/1
  PS-Simulink Converter6/1 -> MATLAB Function/1(xa)
  PS-Simulink Converter7/1 -> MATLAB Function/2(ya)
  PS-Simulink Converter8/1 -> MATLAB Function/3(xb)
  PS-Simulink Converter9/1 -> MATLAB Function/4(yb)
  Unwrap/1 -> [theta]
  MATLAB Function/1(y) -> Unwrap/1
  Repeating Sequence Interpolated/1 -> [phi_1], Gain6/1
  Repeating Sequence Interpolated1/1 -> [phi_2], Gain8/1
  Repeating Sequence Interpolated3/1 -> [phi_3], Gain7/1
  Repeating Sequence Interpolated2/1 -> [phi_4], Gain9/1
  [phi_1] -> Mux/1
  [phi_2] -> Mux/2
  [phi_3] -> Mux/3
  [phi_4] -> Mux/4
  connections:
  Bateria_1_RIGID/LConn1 -- Bateria_Soporte_Sup_1_RIGID/RConn1
  front_wheel/LConn1 -- front_spherical/RConn1
  REAR_chasis/LConn1 -- rear_female/RConn1
  FRONT_chasis/LConn2 -- front_female/RConn1
  Weld Joint1/LConn1 -- rear_male/RConn1
  Weld Joint1/RConn1 -- front_female/LConn1
  Revolute Joint8/LConn1 -- rear_right_wheel/RConn3
  Revolute Joint7/LConn1 -- rear_right_wheel/RConn2
  Revolute Joint6/LConn1 -- rear_right_wheel/RConn1
  front_left_cover/LConn1 -- front_left_wheel/LConn1
  Revolute Joint17/LConn1 -- front_left_wheel/RConn6
  Revolute Joint16/LConn1 -- front_left_wheel/RConn5
  Revolute Joint15/LConn1 -- front_left_wheel/RConn4
  Revolute Joint14/LConn1 -- front_left_wheel/RConn3
  Revolute Joint13/LConn1 -- front_left_wheel/RConn2
  Revolute Joint12/LConn1 -- front_left_wheel/RConn1
  rear_right_wheel/LConn1 -- RI_tapa_2_2_RIGID/LConn1
  front_left_couple/RConn1 -- front_left_wheel/LConn2
  pin/LConn1 -- Mecanismo_Servo_1_RIGID/RConn1
  pin/RConn1 -- Mecanismo_Brazo_1_RIGID/LConn1
  front_servo/RConn1 -- front_servo_act/LConn1
  front_arm/LConn1 -- front_servo_act/RConn1
  REAR_chasis/RConn3 -- Mecanismo_Cubierta_Servo_1_RIGID/LConn1
  Mecanismo_Cubierta_Servo_1_RIGID/RConn1 -- Mecanismo_Servo_1_RIGID/LConn1
  FRONT_chasis/RConn4 -- front_servo_support/LConn1
  front_servo_support/RConn1 -- front_servo/LConn1
  Bateria_Soporte_Sup_1_RIGID/LConn1 -- rear_battery_support/RConn1
  Cople_1_RIGID/RConn1 -- rear_right_wheel/LConn2
  Bateria_Soporte_Sup_1_RIGID/LConn2 -- cubierta_superior_1_RIGID/LConn1
  Bateria_Soporte_Sup_3_RIGID/LConn1 -- Bateria_soporte_Inf_1_3_RIGID/RConn1
  Bateria_Soporte_Sup_3_RIGID/RConn1 -- front_main_frame/LConn1
  REAR_chasis/LConn5 -- rear_battery_supppor/RConn1
  REAR_chasis/RConn2 -- rear_male/LConn2
  REAR_chasis/RConn4 -- Base_Soporte_Motor_1_RIGID/LConn1
  REAR_chasis/RConn1 -- Base_Soporte_Motor_2_RIGID/LConn1
  FRONT_chasis/RConn2 -- Bateria_soporte_Inf_1_3_RIGID/LConn1
  FRONT_chasis/LConn3 -- front_battery_support/RConn1
  Revolute Joint11/LConn1 -- rear_right_wheel/RConn6
  FRONT_chasis/RConn3 -- front_male/RConn1
  FRONT_chasis/RConn5 -- front_rigth_motor_support/LConn1
  RD_Tapa_2_1_RIGID/LConn1 -- RD_Tapa_2_2_RIGID/LConn1
  Revolute Joint5/LConn1 -- RD_Tapa_2_1_RIGID/RConn6
  Rodillo_10_RIGID/LConn1 -- Revolute Joint5/RConn1
  Revolute Joint4/LConn1 -- RD_Tapa_2_1_RIGID/RConn5
  Revolute Joint3/LConn1 -- RD_Tapa_2_1_RIGID/RConn4
  Revolute Joint2/LConn1 -- RD_Tapa_2_1_RIGID/RConn3
  Cople_3_RIGID/RConn1 -- RD_Tapa_2_1_RIGID/LConn2
  Revolute Joint1/LConn1 -- RD_Tapa_2_1_RIGID/RConn2
  Revolute Joint/LConn1 -- RD_Tapa_2_1_RIGID/RConn1
  RD_Tapa_2_5_RIGID/LConn1 -- RD_Tapa_2_6_RIGID/LConn1
  Revolute Joint23/LConn1 -- RD_Tapa_2_6_RIGID/RConn6
  Revolute Joint10/LConn1 -- rear_right_wheel/RConn5
  Revolute Joint22/LConn1 -- RD_Tapa_2_6_RIGID/RConn5
  Revolute Joint21/LConn1 -- RD_Tapa_2_6_RIGID/RConn4
  Revolute Joint20/LConn1 -- RD_Tapa_2_6_RIGID/RConn3
  Revolute Joint19/LConn1 -- RD_Tapa_2_6_RIGID/RConn2
  Revolute Joint18/LConn1 -- RD_Tapa_2_6_RIGID/RConn1
  Cople_7_RIGID/RConn1 -- RD_Tapa_2_6_RIGID/LConn2
  joint_4/LConn1 -- Base_Motor_1_RIGID/RConn1
  joint_4/RConn1 -- Cople_1_RIGID/LConn1
  joint_3/LConn1 -- Base_Motor_2_RIGID/RConn1
  joint_3/RConn1 -- Cople_3_RIGID/LConn1
  joint_1/LConn1 -- Base_Motor_6_RIGID/RConn1
  joint_1/RConn1 -- front_left_couple/LConn1
  joint_2/LConn1 -- front_right_motor/RConn1
  joint_2/RConn1 -- Cople_7_RIGID/LConn1
  Mecanismo_Brazo_1_RIGID/RConn1 -- Mecanismo_Espaciador_1_RIGID/LConn1
  Revolute Joint9/LConn1 -- rear_right_wheel/RConn4
  Mecanismo_Espaciador_1_RIGID/RConn1 -- Mecanismo_Rptula_1_RIGID/LConn1
  front_arm/RConn1 -- Front_spacer/LConn1
  Front_spacer/RConn1 -- front_joint_ball/LConn1
  Base_Motor_1_RIGID/LConn1 -- Base_Soporte_Motor_1_RIGID/RConn1
  Base_Motor_2_RIGID/LConn1 -- Base_Soporte_Motor_2_RIGID/RConn1
  front_right_motor/LConn1 -- front_rigth_motor_support/RConn1
  Base_Motor_6_RIGID/LConn1 -- Front_support_motor/RConn1
  Mecanismo_Rptula_1_RIGID/RConn1 -- Spherical/LConn1
  Mecanismo_Rueda_1_RIGID/LConn1 -- Spherical/RConn1
  front_joint_ball/RConn1 -- front_spherical/LConn1
  Bateria_Soporte_Sup_3_RIGID/RConn2 -- front_battery/LConn1
  Front_support_motor/LConn1 -- FRONT_chasis/RConn1
  rear_battery_support/LConn1 -- REAR_chasis/LConn4
  Revolute Joint/RConn1 -- Rodillo_9_RIGID/LConn1
  Revolute Joint1/RConn1 -- Rodillo_8_RIGID/LConn1
  Revolute Joint2/RConn1 -- Rodillo_13_RIGID/LConn1
  Revolute Joint3/RConn1 -- Rodillo_12_RIGID/LConn1
  Revolute Joint4/RConn1 -- Rodillo_11_RIGID/LConn1
  Revolute Joint11/RConn1 -- Rodillo_2_RIGID/LConn1
  Revolute Joint10/RConn1 -- Rodillo_3_RIGID/LConn1
  Revolute Joint9/RConn1 -- Rodillo_4_RIGID/LConn1
  Revolute Joint8/RConn1 -- Rodillo_5_RIGID/LConn1
  Revolute Joint6/RConn1 -- Rodillo_7_RIGID/LConn1
  Revolute Joint7/RConn1 -- Rodillo_6_RIGID/LConn1
  Revolute Joint23/RConn1 -- Rodillo_33_RIGID/LConn1
  Revolute Joint22/RConn1 -- Rodillo_34_RIGID/LConn1
  Revolute Joint21/RConn1 -- Rodillo_35_RIGID/LConn1
  Revolute Joint20/RConn1 -- Rodillo_36_RIGID/LConn1
  Revolute Joint19/RConn1 -- Rodillo_37_RIGID/LConn1
  Revolute Joint18/RConn1 -- Rodillo_38_RIGID/LConn1
  Revolute Joint12/RConn1 -- Rodillo_31_RIGID/LConn1
  Revolute Joint13/RConn1 -- Rodillo_30_RIGID/LConn1
  Revolute Joint14/RConn1 -- Rodillo_29_RIGID/LConn1
  Revolute Joint15/RConn1 -- Rodillo_28_RIGID/LConn1
  Revolute Joint16/RConn1 -- Rodillo_27_RIGID/LConn1
  Revolute Joint17/RConn1 -- Rodillo_26_RIGID/LConn1
  Rodillo_9_RIGID/RConn1 -- Spatial Contact Force/LConn1
  Rodillo_8_RIGID/RConn1 -- Spatial Contact Force1/LConn1
  Rodillo_13_RIGID/RConn1 -- Spatial Contact Force2/LConn1
  Rodillo_12_RIGID/RConn1 -- Spatial Contact Force3/LConn1
  Rodillo_11_RIGID/RConn1 -- Spatial Contact Force4/LConn1
  Rodillo_10_RIGID/RConn1 -- Spatial Contact Force5/LConn1
  Rodillo_7_RIGID/RConn1 -- Spatial Contact Force6/LConn1
  Rodillo_2_RIGID/RConn1 -- Spatial Contact Force11/LConn1
  Rodillo_3_RIGID/RConn1 -- Spatial Contact Force10/LConn1
  Rodillo_4_RIGID/RConn1 -- Spatial Contact Force9/LConn1
  Rodillo_5_RIGID/RConn1 -- Spatial Contact Force8/LConn1
  Rodillo_6_RIGID/RConn1 -- Spatial Contact Force7/LConn1
  Rodillo_31_RIGID/RConn1 -- Spatial Contact Force20/LConn1
  Rodillo_30_RIGID/RConn1 -- Spatial Contact Force21/LConn1
  Rodillo_38_RIGID/RConn1 -- Spatial Contact Force14/LConn1
  Rodillo_37_RIGID/RConn1 -- Spatial Contact Force15/LConn1
  Rodillo_33_RIGID/RConn1 -- Spatial Contact Force13/LConn1
  Rodillo_34_RIGID/RConn1 -- Spatial Contact Force12/LConn1
  Rodillo_35_RIGID/RConn1 -- Spatial Contact Force17/LConn1
  Rodillo_36_RIGID/RConn1 -- Spatial Contact Force16/LConn1
  Rodillo_29_RIGID/RConn1 -- Spatial Contact Force22/LConn1
  Rodillo_28_RIGID/RConn1 -- Spatial Contact Force23/LConn1
  Rodillo_27_RIGID/RConn1 -- Spatial Contact Force18/LConn1
  Rodillo_26_RIGID/RConn1 -- Spatial Contact Force19/LConn1
  joint_1/LConn2 -- Simulink-PS Converter/RConn1
  joint_2/LConn2 -- Simulink-PS Converter1/RConn1
  Simulink-PS Converter3/RConn1 -- joint_3/LConn2
  joint_4/LConn2 -- Simulink-PS Converter4/RConn1
  Simulink-PS Converter2/RConn1 -- pin/LConn2
  front_servo_act/LConn2 -- Simulink-PS Converter5/RConn1
  Transform Sensor/LConn1 -- Transform Sensor1/LConn1 -- Rigid Transform2/RConn1 -- REFERENCE/RConn1
  Transform Sensor/RConn3 -- PS-Simulink Converter5/LConn1
  Transform Sensor/RConn2 -- PS-Simulink Converter4/LConn1
  Transform Sensor/RConn5 -- PS-Simulink Converter7/LConn1 -- PS-Simulink Converter3/LConn1
  Transform Sensor/RConn7 -- PS-Simulink Converter2/LConn1
  Rigid Transform/RConn1 -- Rigid Transform1/LConn1
  Transform Sensor/RConn4 -- PS-Simulink Converter6/LConn1 -- PS-Simulink Converter/LConn1
  Transform Sensor/RConn6 -- PS-Simulink Converter1/LConn1
  REAR_chasis/LConn3 -- SixDOF1/RConn1
  Rigid Transform1/RConn1 -- Rigid Transform2/LConn1
  MechanismConfiguration/RConn1 -- World/RConn1 -- Rigid Transform/LConn1 -- Solver Configuration1/RConn1 -- SixDOF1/LConn1 -- Rigid Transform3/LConn1
  Rigid Transform3/RConn1 -- Brick Solid/RConn1
  Brick Solid/LConn1 -- Spatial Contact Force20/RConn1 -- Spatial Contact Force21/RConn1 -- Spatial Contact Force22/RConn1 -- Spatial Contact Force23/RConn1 -- Spatial Contact Force18/RConn1 -- Spatial Contact Force12/RConn1 -- Spatial Contact Force13/RConn1 -- Spatial Contact Force17/RConn1 -- Spatial Contact Force16/RConn1 -- Spatial Contact Force15/RConn1 -- Spatial Contact Force14/RConn1 -- Spatial Contact Force19/RConn1 -- Spatial Contact Force/RConn1 -- Spatial Contact Force1/RConn1 -- Spatial Contact Force2/RConn1 -- Spatial Contact Force3/RConn1 -- Spatial Contact Force10/RConn1 -- Spatial Contact Force11/RConn1 -- Spatial Contact Force9/RConn1 -- Spatial Contact Force8/RConn1 -- Spatial Contact Force7/RConn1 -- Spatial Contact Force6/RConn1 -- Spatial Contact Force5/RConn1 -- Spatial Contact Force4/RConn1
  PS-Simulink Converter8/LConn1 -- Transform Sensor1/RConn2
  PS-Simulink Converter9/LConn1 -- Transform Sensor1/RConn3
  Transform Sensor1/RConn1 -- FRONT_chasis/LConn4
  Transform Sensor/RConn1 -- REAR_chasis/LConn2
